simulink model "modele_dynamiczne"  (R2021a)
settings: Solver=VariableStepAuto  StartTime=0.0  StopTime=60  RelTol=1e-3
values from neighbouring files (symbols this model uses):
  a1 = 0.32    [Wartosci_w_zadaniu.m]    (also in zad_4.m)
  a2 = 0.45    [Wartosci_w_zadaniu.m]    (also in zad_4.m)
  a3 = -0.29    [Wartosci_w_zadaniu.m]    (also in zad_4.m)
  a4 = -0.1    [Wartosci_w_zadaniu.m]    (also in zad_4.m)
  K = 2    [Wartosci_w_zadaniu.m]    (also in zad_4.m)
  T = 1.5    [zad_4.m]
  T1 = 5    [Wartosci_w_zadaniu.m]    (also in zad_4.m)
  T2 = 8    [Wartosci_w_zadaniu.m]    (also in zad_4.m)
settings Model: Creator=ADMIN  LastModifiedBy=ADMIN

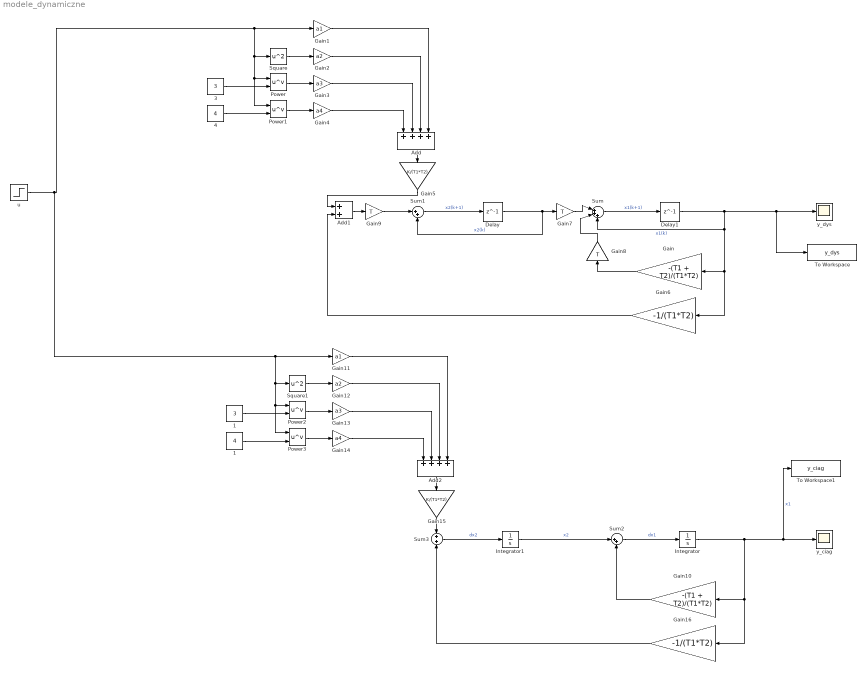
== system modele_dynamiczne ==
  " 1" : Constant  Value=3
  " 3" : Constant  Value=3
  1 : Constant  Value=4
  4 : Constant  Value=4
  Add : Sum  Inputs=++++
  Add1 : Sum
  Add2 : Sum  Inputs=++++
  Delay : Delay  DelayLength=1  InitialCondition=0  SampleTime=T
  Delay1 : Delay  DelayLength=1  InitialCondition=0  SampleTime=T
  Gain : Gain  Gain=-(T1 + T2)/(T1*T2)
  Gain1 : Gain  Gain=a1
  Gain10 : Gain  Gain=-(T1 + T2)/(T1*T2)
  Gain11 : Gain  Gain=a1
  Gain12 : Gain  Gain=a2
  Gain13 : Gain  Gain=a3
  Gain14 : Gain  Gain=a4
  Gain15 : Gain  Gain=K/(T1*T2)
  Gain16 : Gain  Gain=-1/(T1*T2)
  Gain2 : Gain  Gain=a2
  Gain3 : Gain  Gain=a3
  Gain4 : Gain  Gain=a4
  Gain5 : Gain  Gain=K/(T1*T2)
  Gain6 : Gain  Gain=-1/(T1*T2)
  Gain7 : Gain  Gain=T
  Gain8 : Gain  Gain=T
  Gain9 : Gain  Gain=T
  Integrator : Integrator
  Integrator1 : Integrator
  Power{,1..3} (4 alike) : Math  Operator=pow  SaturateOnIntegerOverflow=on
  Square : Math  Operator=square  SaturateOnIntegerOverflow=on
  Square1 : Math  Operator=square  SaturateOnIntegerOverflow=on
  Sum : Sum  Inputs=|+++
  Sum1 : Sum  Inputs=|++
  Sum2 : Sum  Inputs=|++
  Sum3 : Sum
  To Workspace : ToWorkspace  VariableName=y_dys  SaveFormat=Structure With Time  SampleTime=T
  To Workspace1 : ToWorkspace  VariableName=y_ciag  SaveFormat=Structure With Time  SampleTime=-1
  u : Step  SampleTime=0
  y_ciag : Scope
  y_dys : Scope
  wires:
  Power1/1 -> Gain4/1
  Gain9/1 -> Sum1/1
  Sum/1 -> Delay1/1  "x1(k+1)"
  Delay1/1 -> Sum/3, Gain6/1, Gain/1, To Workspace/1, y_dys/1  "x1(k)"
  Gain8/1 -> Sum/2
  Gain/1 -> Gain8/1
  Delay/1 -> Sum1/2, Gain7/1  "x2(k)"
  Gain4/1 -> Add/1
  Gain3/1 -> Add/2
  4/1 -> Power1/2
  " 3"/1 -> Power/2
  Gain5/1 -> Add1/1
  u/1 -> Power3/1, Power2/1, Square1/1, Gain11/1, Power1/1, Power/1, Square/1, Gain1/1
  Gain7/1 -> Sum/1
  Gain1/1 -> Add/4
  Gain2/1 -> Add/3
  Add/1 -> Gain5/1
  Square/1 -> Gain2/1
  Add1/1 -> Gain9/1
  Gain6/1 -> Add1/2
  Sum1/1 -> Delay/1  "x2(k+1)"
  Power/1 -> Gain3/1
  Gain10/1 -> Sum2/2
  Square1/1 -> Gain12/1
  Gain11/1 -> Add2/4
  Gain13/1 -> Add2/2
  Add2/1 -> Gain15/1
  Integrator/1 -> Gain16/1, Gain10/1, To Workspace1/1, y_ciag/1  "x1"
  Gain15/1 -> Sum3/1
  Sum2/1 -> Integrator/1  "dx1"
  Sum3/1 -> Integrator1/1  "dx2"
  Power2/1 -> Gain13/1
  Integrator1/1 -> Sum2/1  "x2"
  Gain12/1 -> Add2/3
  " 1"/1 -> Power2/2
  Gain14/1 -> Add2/1
  Power3/1 -> Gain14/1
  1/1 -> Power3/2
  Gain16/1 -> Sum3/2
